simulink model "Hydrogen_platform"  (R2024b)
settings: Solver=VariableStepAuto  StartTime=0.0  StopTime=10.0  FixedStep=0.001  RelTol=1e-3
(part 1 of 2)
settings Model: Creator=Administrator  LastModifiedBy=wangx
settings OptimizationCC: DefaultParameterBehavior=Inlined  EnhancedBackFolding=on  PassReuseOutputArgsAs=Individual arguments  ZeroExternalMemoryAtStartup=off  ZeroInternalMemoryAtStartup=off  OptimizeBlockOrder=speed  DifferentSizesBufferReuse=on  OptimizationCustomize=off  EfficientTunableParamExpr=on
settings DebuggingCC: ParameterTunabilityLossMsg=error  ForceCombineOutputUpdateInSim=on
settings HardwareCC: TargetBitPerPointer=64  TargetBitPerSizeT=64  TargetBitPerPtrDiffT=64  TargetLongLongMode=on  TargetIntDivRoundTo=Zero  TargetEndianess=LittleEndian  TargetWordSize=64  TargetHWDeviceType=MATLAB Host  ProdEqTarget=off
settings ModelReferenceCC: EnableRefExpFcnMdlSchedulingChecks=on
settings SFSimCC: MATLABDynamicMemAlloc=off
settings RTWCC: Description=Embedded Coder  SystemTargetFile=ert.tlc  TemplateMakefile=ert_default_tmf  GPUComputeCapability=3.5
settings CodeAppCC: ForceParamTrailComments=on  IgnoreCustomStorageClasses=off  OperatorAnnotations=on  SimulinkDataObjDesc=on  SFDataObjDesc=on  InsertBlockDesc=on
settings ERTTargetCC: TargetLangStandard=C99 (ISO)  GenerateSampleERTMain=on  SupportContinuousTime=on  ERTCustomFileTemplate=example_file_process.tlc  DynamicArrayContainerType=coder::array

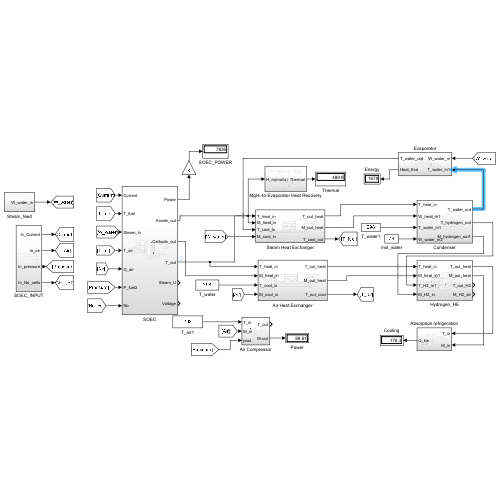
[thumbnail: Simulink's stored preview of the top-level diagram]
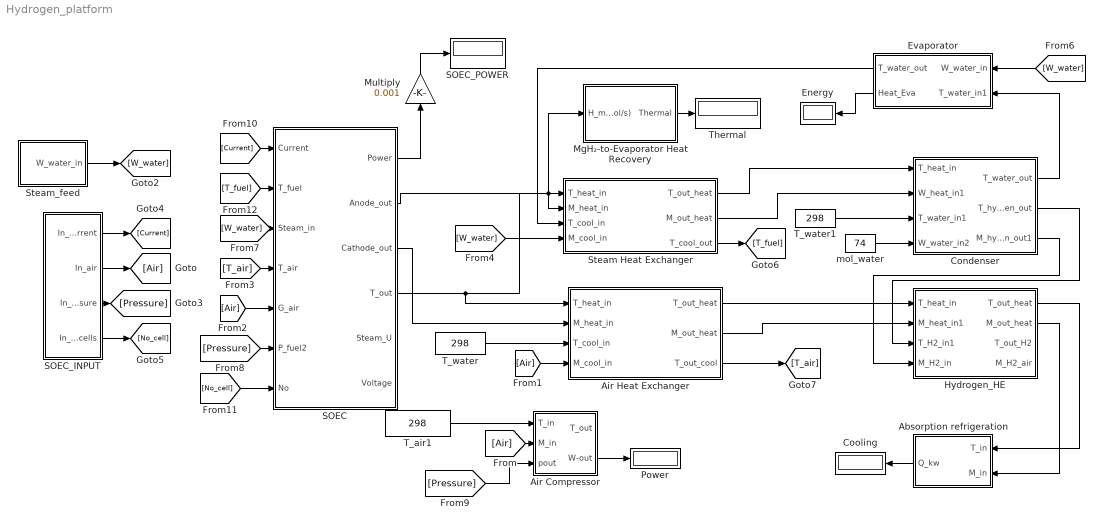
== system Hydrogen_platform ==
  Absorption refrigeration : Subsystem
  Air Compressor : Subsystem
  Air Heat Exchanger : Subsystem
  Condenser : Subsystem
  Cooling : Display
  Energy : Display
  Evaporator : Subsystem
  Hydrogen_HE : Subsystem
  MgH₂-to-Evaporator Heat Recovery : Subsystem
  Multiply : Gain  Gain=0.001
  Power : Display
  SOEC : Subsystem
  SOEC_INPUT : Subsystem
  SOEC_POWER : Display
  Steam Heat Exchanger : Subsystem
  Steam_feed : Subsystem
  T_air1 : Constant  Value=298
  T_water : Constant  Value=298
  T_water1 : Constant  Value=298
  Thermal : Display
  mol_water : Constant  Value=74
  wires:
  mol_water/1 -> Condenser/4(W_water_in2)
  SOEC/3(Cathode_out) -> Air Heat Exchanger/2(M_heat_in)
  T_air1/1 -> Air Compressor/1(T_in)
  SOEC/4(T_out) -> Steam Heat Exchanger/1(T_heat_in), Air Heat Exchanger/1(T_heat_in)
  Evaporator/1(T_water_out) -> Steam Heat Exchanger/3(T_cool_in)
  Condenser/1(T_water_out) -> Evaporator/2(T_water_in1)
  SOEC/2(Anode_out) -> MgH₂-to-Evaporator Heat Recovery/1(H_m(mol/s)), Steam Heat Exchanger/2(M_heat_in)
  [Air] -> Air Compressor/2(M_in)
  [Air] -> SOEC/5(G_air)
  SOEC_INPUT/2(In_air) -> [Air]
  [T_air] -> SOEC/4(T_air)
  [W_water] -> Steam Heat Exchanger/4(M_cool_in)
  Steam_feed/1(W_water_in) -> [W_water]
  [W_water] -> SOEC/3(Steam_in)
  SOEC_INPUT/3(In_pressure) -> [Pressure]
  [Pressure] -> SOEC/6(P_fuel2)
  [Pressure] -> Air Compressor/3(pout)
  SOEC_INPUT/1(In_Current) -> [Current]
  [Current] -> SOEC/1(Current)
  [No_cell] -> SOEC/7(No)
  SOEC_INPUT/4(In_No_cells) -> [No_cell]
  [T_fuel] -> SOEC/2(T_fuel)
  T_water1/1 -> Condenser/3(T_water_in1)
  Condenser/2(T_hydrogen_out) -> Hydrogen_HE/3(T_H2_in1)
  Condenser/3(M_hydrogen_out1) -> Hydrogen_HE/4(M_H2_in)
  Hydrogen_HE/1(T_out_heat) -> Absorption refrigeration/1(T_in)
  Hydrogen_HE/2(M_out_heat) -> Absorption refrigeration/2(M_in)
  Multiply/1 -> SOEC_POWER/1
  SOEC/1(Power) -> Multiply/1
  Evaporator/2(Heat_Eva) -> Energy/1
  Air Compressor/2(W-out) -> Power/1
  Steam Heat Exchanger/1(T_out_heat) -> Condenser/1(T_heat_in)
  Steam Heat Exchanger/2(M_out_heat) -> Condenser/2(W_heat_in1)
  Steam Heat Exchanger/3(T_cool_out) -> [T_fuel]
  [Air] -> Air Heat Exchanger/4(M_cool_in)
  T_water/1 -> Air Heat Exchanger/3(T_cool_in)
  Air Heat Exchanger/3(T_out_cool) -> [T_air]
  Air Heat Exchanger/1(T_out_heat) -> Hydrogen_HE/1(T_heat_in)
  Air Heat Exchanger/2(M_out_heat) -> Hydrogen_HE/2(M_heat_in1)
  [W_water] -> Evaporator/1(W_water_in)
  Absorption refrigeration/1(Q_kw) -> Cooling/1
  MgH₂-to-Evaporator Heat Recovery/1(Thermal) -> Thermal/1

== system Hydrogen_platform/Absorption refrigeration ==
  T_in : Inport
  M_in : Inport  Port=2
  Add : Sum  Inputs=-+
  Cop : Constant  Value=1.3
  Demux : Demux  Outputs=2
  Divide : Product  Inputs=**
  Energy : Product  Inputs=***
  Energy1 : Product  Inputs=***
  T_out : Constant  Value=273+120
  air_out1 : Subsystem
  air_out2 : Subsystem
  kW : Gain  Gain=0.001
  sum : Fcn  Expr=u(1)+u(2)
  Q_kw : Outport
  wires:
  M_in/1 -> sum/1, Demux/1
  Demux/1 -> air_out2/2(O2), air_out1/2(O2)
  Demux/2 -> air_out2/3(N2), air_out1/3(N2)
  T_in/1 -> Energy/2, air_out2/1(T_cool_out)
  air_out2/1(C_p) -> Energy/3
  Energy/1 -> Add/2
  sum/1 -> Energy1/2, Energy/1
  T_out/1 -> Energy1/1, air_out1/1(T_cool_out)
  air_out1/1(C_p) -> Energy1/3
  Energy1/1 -> Add/1
  Add/1 -> Divide/1
  Cop/1 -> Divide/2
  Divide/1 -> kW/1
  kW/1 -> Q_kw/1

== system Hydrogen_platform/Air Compressor ==
  T_in : Inport
  M_in : Inport  Port=2
  pout : Inport  Port=3
  Add : Sum  Inputs=+-
  Gain : Gain  Gain=1e-5
  Gain1 : Gain  Gain=0.21
  Gain2 : Gain  Gain=0.79
  Gain3 : Gain  Gain=0.001
  Mux : Mux  Inputs=2
  Product : Product
  Product1 : Product
  Product2 : Product
  T_jisuan : Fcn  Expr=u(1)*(1+(1/0.85)*(u(2)^0.285-1))
  air_out1 : Subsystem
  air_out3 : Subsystem
  T_out : Outport
  W-out : Outport  Port=2
  wires:
  T_jisuan/1 -> air_out1/1(T_cool_out), T_out/1, Product1/1
  Mux/1 -> T_jisuan/1
  T_in/1 -> air_out3/1(T_cool_out), Product/1, Mux/1
  pout/1 -> Gain/1
  Gain/1 -> Mux/2
  M_in/1 -> Product2/2, Gain2/1, Gain1/1
  Gain1/1 -> air_out1/2(O2), air_out3/2(O2)
  Gain2/1 -> air_out3/3(N2), air_out1/3(N2)
  air_out3/1(C_p) -> Product/2
  air_out1/1(C_p) -> Product1/2
  Product1/1 -> Add/1
  Product/1 -> Add/2
  Product2/1 -> Gain3/1
  Add/1 -> Product2/1
  Gain3/1 -> W-out/1

== system Hydrogen_platform/Air Heat Exchanger ==
  T_heat_in : Inport
  M_heat_in : Inport  Port=2
  T_cool_in : Inport  Port=3
  M_cool_in : Inport  Port=4
  First_Air_HE : Subsystem
  Second_Air_HE : Subsystem
  T_out_heat : Outport
  M_out_heat : Outport  Port=2
  T_out_cool : Outport  Port=3
  wires:
  First_Air_HE/1(T_out_heat) -> Second_Air_HE/1(T_heat_in)
  First_Air_HE/2(M_out_heat) -> Second_Air_HE/2(M_heat_in1)
  Second_Air_HE/3(T_out_cool) -> First_Air_HE/3(T_cool_in1)
  Second_Air_HE/4(M_out_cool) -> First_Air_HE/4(M_cool_in)
  M_cool_in/1 -> Second_Air_HE/4(M_cool_in)
  First_Air_HE/3(T_out_cool) -> T_out_cool/1
  T_cool_in/1 -> Second_Air_HE/3(T_cool_in1)
  T_heat_in/1 -> First_Air_HE/1(T_heat_in)
  M_heat_in/1 -> First_Air_HE/2(M_heat_in1)
  Second_Air_HE/1(T_out_heat) -> T_out_heat/1
  Second_Air_HE/2(M_out_heat) -> M_out_heat/1

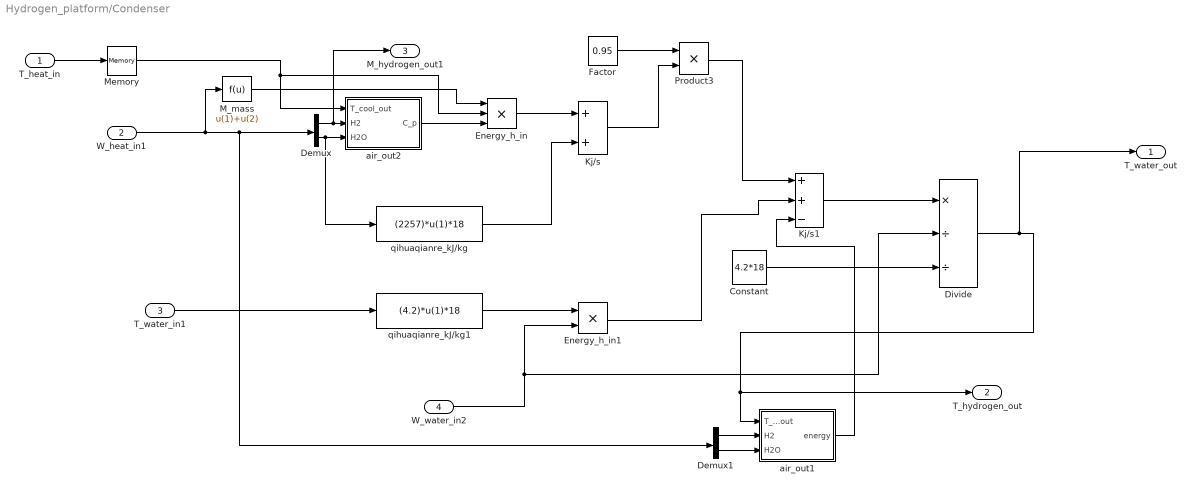
== system Hydrogen_platform/Condenser ==
  T_heat_in : Inport
  W_heat_in1 : Inport  Port=2
  T_water_in1 : Inport  Port=3
  W_water_in2 : Inport  Port=4
  Constant : Constant  Value=4.2*18
  Demux : Demux  Outputs=2
  Demux1 : Demux  Outputs=2
  Divide : Product  Inputs=*//
  Energy_h_in : Product  Inputs=3
  Energy_h_in1 : Product
  Factor : Constant  Value=0.95
  Kj/s : Sum
  Kj/s1 : Sum  Inputs=++-
  M_mass : Fcn  Expr=u(1)+u(2)
  Memory : Memory  InitialCondition=500
  Product3 : Product
  air_out1 : Subsystem
  air_out2 : Subsystem
  qihuaqianre_kJ/kg : Fcn  Expr=(2257)*u(1)*18
  qihuaqianre_kJ/kg1 : Fcn  Expr=(4.2)*u(1)*18
  T_water_out : Outport
  T_hydrogen_out : Outport  Port=2
  M_hydrogen_out1 : Outport  Port=3
  wires:
  Demux/1 -> M_hydrogen_out1/1, air_out2/2(H2)
  Demux/2 -> qihuaqianre_kJ/kg/1, air_out2/3(H2O)
  W_heat_in1/1 -> M_mass/1, Demux/1, Demux1/1
  T_heat_in/1 -> Memory/1
  air_out2/1(C_p) -> Energy_h_in/3
  M_mass/1 -> Energy_h_in/1
  Energy_h_in/1 -> Kj/s/1
  Factor/1 -> Product3/1
  Kj/s/1 -> Product3/2
  qihuaqianre_kJ/kg/1 -> Kj/s/2
  T_water_in1/1 -> qihuaqianre_kJ/kg1/1
  qihuaqianre_kJ/kg1/1 -> Energy_h_in1/1
  W_water_in2/1 -> Divide/2, Energy_h_in1/2
  Product3/1 -> Kj/s1/1
  Energy_h_in1/1 -> Kj/s1/2
  Constant/1 -> Divide/3
  Divide/1 -> T_water_out/1, air_out1/1(T_cool_out), T_hydrogen_out/1
  Demux1/1 -> air_out1/2(H2)
  Demux1/2 -> air_out1/3(H2O)
  air_out1/1(energy) -> Kj/s1/3
  Kj/s1/1 -> Divide/1
  Memory/1 -> air_out2/1(T_cool_out), Energy_h_in/2

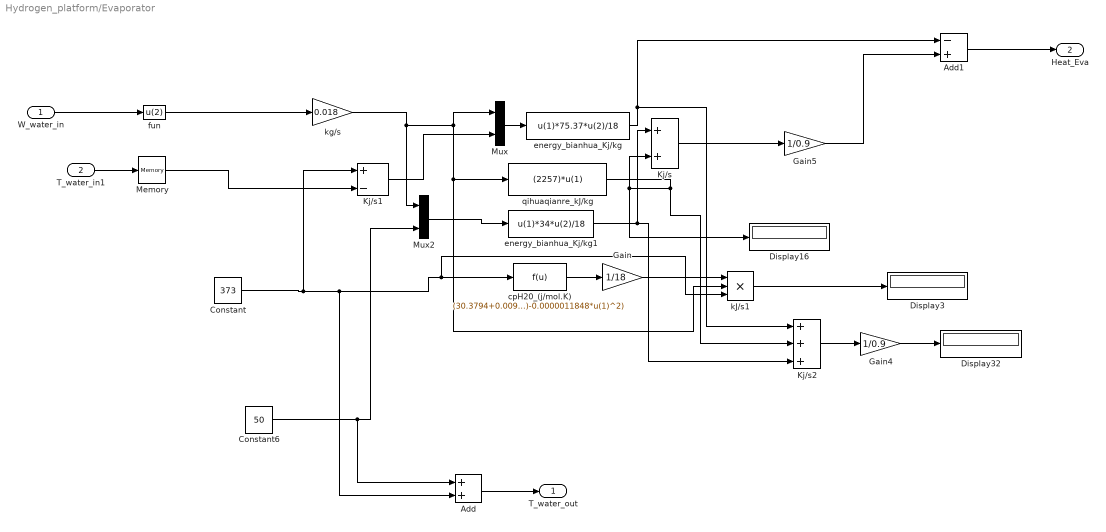
== system Hydrogen_platform/Evaporator ==
  W_water_in : Inport
  T_water_in1 : Inport  Port=2
  Add : Sum
  Add1 : Sum  Inputs=-+
  Constant : Constant  Value=373
  Constant6 : Constant  Value=50
  Display16 : Display
  Display3 : Display
  Display32 : Display
  Gain : Gain  Gain=1/18
  Gain4 : Gain  Gain=1/0.9
  Gain5 : Gain  Gain=1/0.9
  Kj/s : Sum
  Kj/s1 : Sum  Inputs=+-
  Kj/s2 : Sum  Inputs=+++
  Memory : Memory  InitialCondition=300
  Mux : Mux  Inputs=2
  Mux2 : Mux  Inputs=2
  cpH20_(j/mol.K) : Fcn  Expr=(30.3794+0.0096212*u(1)-0.0000011848*u(1)^2)
  energy_bianhua_Kj/kg : Fcn  Expr=u(1)*75.37*u(2)/18
  energy_bianhua_Kj/kg1 : Fcn  Expr=u(1)*34*u(2)/18
  fun : Fcn  Expr=u(2)
  kJ/s1 : Product  Inputs=3
  kg/s : Gain  Gain=0.018
  qihuaqianre_kJ/kg : Fcn  Expr=(2257)*u(1)
  T_water_out : Outport
  Heat_Eva : Outport  Port=2
  wires:
  W_water_in/1 -> fun/1
  energy_bianhua_Kj/kg/1 -> Kj/s2/1, Add1/1
  qihuaqianre_kJ/kg/1 -> Kj/s2/2, Kj/s/2, Display16/1
  Constant/1 -> kJ/s1/3, cpH20_(j/mol.K)/1, Add/2, Kj/s1/1
  cpH20_(j/mol.K)/1 -> Gain/1
  Gain/1 -> kJ/s1/1
  kJ/s1/1 -> Display3/1
  T_water_in1/1 -> Memory/1
  Mux/1 -> energy_bianhua_Kj/kg/1
  Kj/s1/1 -> Mux/2
  Memory/1 -> Kj/s1/2
  energy_bianhua_Kj/kg1/1 -> Kj/s2/3, Kj/s/1
  kg/s/1 -> Mux2/1, Mux/1, kJ/s1/2, qihuaqianre_kJ/kg/1
  Mux2/1 -> energy_bianhua_Kj/kg1/1
  Constant6/1 -> Add/1, Mux2/2
  Add/1 -> T_water_out/1
  Kj/s/1 -> Gain5/1
  Kj/s2/1 -> Gain4/1
  Gain4/1 -> Display32/1
  Gain5/1 -> Add1/2
  fun/1 -> kg/s/1
  Add1/1 -> Heat_Eva/1

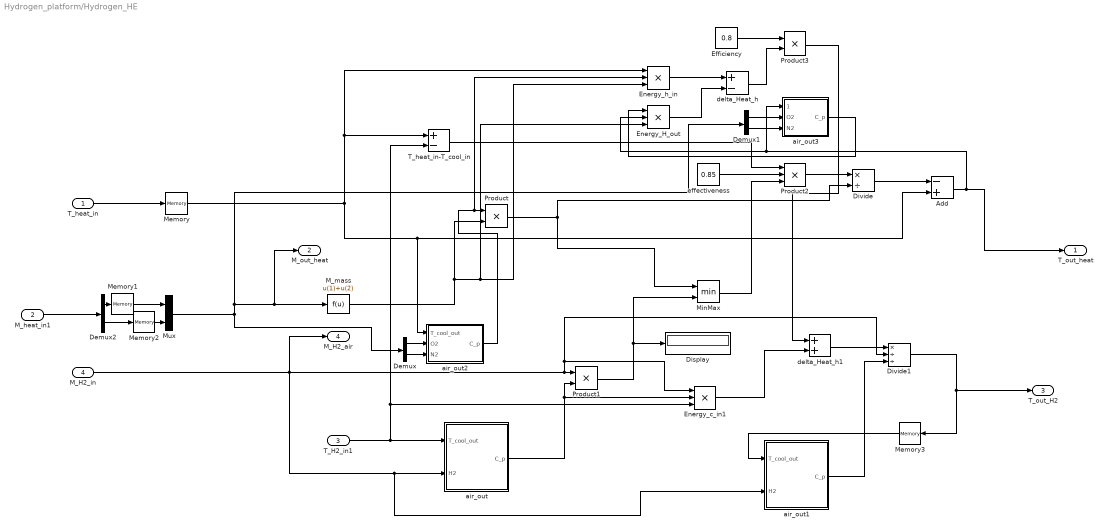
== system Hydrogen_platform/Hydrogen_HE ==
  T_heat_in : Inport
  M_heat_in1 : Inport  Port=2
  T_H2_in1 : Inport  Port=3
  M_H2_in : Inport  Port=4
  Add : Sum  Inputs=-+
  Demux : Demux  Outputs=2
  Demux1 : Demux  Outputs=2
  Demux2 : Demux  Outputs=2
  Display : Display
  Divide : Product  Inputs=*/
  Divide1 : Product  Inputs=*//
  Efficiency : Constant  Value=0.8
  Energy_H_out : Product  Inputs=3
  Energy_c_in1 : Product  Inputs=3
  Energy_h_in : Product  Inputs=3
  M_mass : Fcn  Expr=u(1)+u(2)
  Memory : Memory  InitialCondition=800
  Memory1 : Memory  InitialCondition=3
  Memory2 : Memory  InitialCondition=3
  Memory3 : Memory  InitialCondition=400
  MinMax : MinMax  Inputs=2
  Mux : Mux  Inputs=2
  Product : Product
  Product1 : Product
  Product2 : Product  Inputs=3
  Product3 : Product
  T_heat_in-T_cool_in : Sum  Inputs=+-
  air_out : Subsystem
  air_out1 : Subsystem
  air_out2 : Subsystem
  air_out3 : Subsystem
  delta_Heat_h : Sum  Inputs=+-
  delta_Heat_h1 : Sum
  effectiveness : Constant  Value=0.85
  T_out_heat : Outport
  M_out_heat : Outport  Port=2
  T_out_H2 : Outport  Port=3
  M_H2_air : Outport  Port=4
  wires:
  Mux/1 -> M_out_heat/1, M_mass/1, Demux1/1, Demux/1
  Product2/1 -> Divide/1
  T_heat_in/1 -> Memory/1
  MinMax/1 -> Product2/3
  M_H2_in/1 -> M_H2_air/1, Energy_c_in1/1, Divide1/2, Product1/1, air_out1/2(H2), air_out/2(H2)
  air_out/1(C_p) -> Product1/2, Energy_c_in1/2
  T_H2_in1/1 -> Energy_c_in1/3, T_heat_in-T_cool_in/2, air_out/1(T_cool_out)
  T_heat_in-T_cool_in/1 -> Product2/1
  air_out2/1(C_p) -> Product/1, Energy_h_in/2
  effectiveness/1 -> Product2/2
  Energy_H_out/1 -> delta_Heat_h/2
  Product1/1 -> MinMax/2, Display/1
  Product/1 -> MinMax/1, Divide/2
  Add/1 -> air_out3/1(T_cool_out), Energy_H_out/2, T_out_heat/1
  Divide/1 -> Add/1
  Energy_h_in/1 -> delta_Heat_h/1
  Energy_c_in1/1 -> delta_Heat_h1/2
  delta_Heat_h1/1 -> Divide1/1
  air_out1/1(C_p) -> Divide1/3
  Divide1/1 -> Memory3/1, T_out_H2/1
  delta_Heat_h/1 -> Product3/2
  Product3/1 -> delta_Heat_h1/1
  Efficiency/1 -> Product3/1
  M_mass/1 -> Energy_h_in/3, Energy_H_out/3, Product/2
  Demux/1 -> air_out2/2(O2)
  Demux/2 -> air_out2/3(N2)
  Demux1/1 -> air_out3/2(O2)
  Demux1/2 -> air_out3/3(N2)
  air_out3/1(C_p) -> Energy_H_out/1
  Memory/1 -> Energy_h_in/1, T_heat_in-T_cool_in/1, air_out2/1(T_cool_out), Add/2
  Demux2/2 -> Memory2/1
  Memory2/1 -> Mux/2
  Memory1/1 -> Mux/1
  Demux2/1 -> Memory1/1
  M_heat_in1/1 -> Demux2/1
  Memory3/1 -> air_out1/1(T_cool_out)

== system Hydrogen_platform/MgH₂-to-Evaporator Heat Recovery ==
  H_m(mol/s) : Inport
  Divide : Product  Inputs=*/*
  H2_kg : Fcn  Expr=u(1)*2*3600/1000
  KgH2/Tank : Constant  Value=25
  kWh/tank : Constant  Value=61.18
  kg/hour : Display
  Thermal : Outport
  wires:
  H_m(mol/s)/1 -> H2_kg/1
  H2_kg/1 -> Divide/1, kg/hour/1
  KgH2/Tank/1 -> Divide/2
  kWh/tank/1 -> Divide/3
  Divide/1 -> Thermal/1

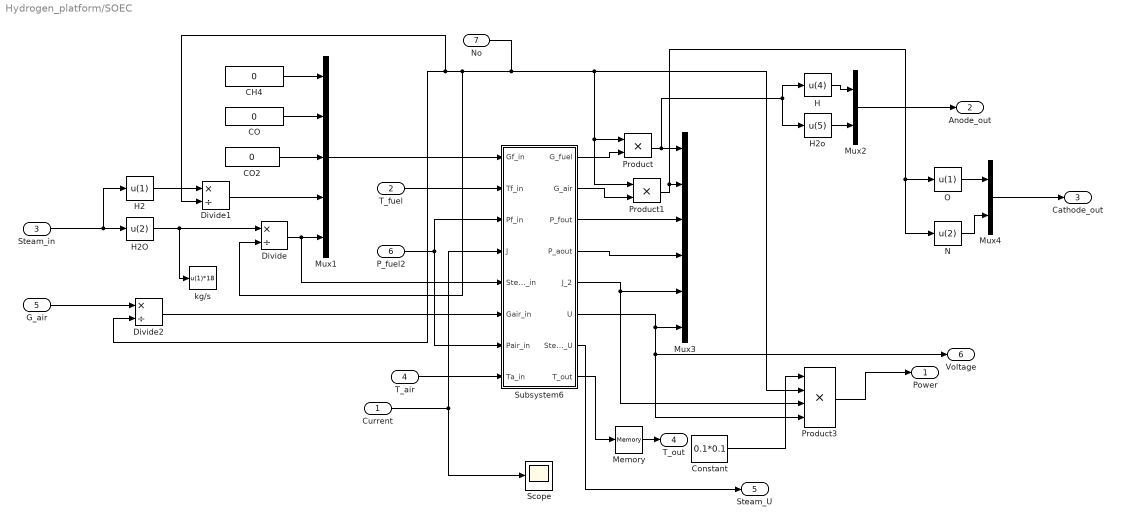
== system Hydrogen_platform/SOEC ==
  Current : Inport
  T_fuel : Inport  Port=2
  Steam_in : Inport  Port=3
  T_air : Inport  Port=4
  G_air : Inport  Port=5
  P_fuel2 : Inport  Port=6
  No : Inport  Port=7
  CH4 : Constant  Value=0
  CO : Constant  Value=0
  CO2 : Constant  Value=0
  Constant : Constant  Value=0.1*0.1
  Divide : Product  Inputs=*/
  Divide1 : Product  Inputs=*/
  Divide2 : Product  Inputs=*/
  H : Fcn  Expr=u(4)
  H2 : Fcn  Expr=u(1)
  H2O : Fcn  Expr=u(2)
  H2o : Fcn  Expr=u(5)
  Memory : Memory  InitialCondition=800
  Mux1 : Mux  Inputs=5
  Mux2 : Mux  Inputs=2
  Mux3 : Mux  Inputs=6
  Mux4 : Mux  Inputs=2
  N : Fcn  Expr=u(2)
  O : Fcn  Expr=u(1)
  Product : Product
  Product1 : Product
  Product3 : Product  Inputs=4
  Scope : Scope
  Subsystem6 : Subsystem
  kg/s : Fcn  Expr=u(1)*18
  Power : Outport
  Anode_out : Outport  Port=2
  Cathode_out : Outport  Port=3
  T_out : Outport  Port=4
  Steam_U : Outport  Port=5
  Voltage : Outport  Port=6
  wires:
  Subsystem6/8(T_out) -> Memory/1
  T_fuel/1 -> Subsystem6/2(Tf_in)
  Current/1 -> Subsystem6/4(J), Scope/1
  Product/1 -> H/1, H2o/1, Mux3/1
  Mux2/1 -> Anode_out/1
  H/1 -> Mux2/1
  Subsystem6/2("\tG_air") -> Product1/2
  No/1 -> Divide2/2, Divide1/2, Divide/2, Product3/2, Product/1, Product1/1
  Subsystem6/5(J_2) -> Mux3/5, Product3/3
  P_fuel2/1 -> Subsystem6/3(Pf_in), Subsystem6/7(Pair_in)
  CO2/1 -> Mux1/3
  Subsystem6/6(U) -> Product3/4, Voltage/1, Mux3/6
  Mux1/1 -> Subsystem6/1(Gf_in)
  Subsystem6/4("\tP_aout") -> Mux3/4
  Product1/1 -> N/1, O/1, Mux3/2
  CH4/1 -> Mux1/1
  CO/1 -> Mux1/2
  H2o/1 -> Mux2/2
  Product3/1 -> Power/1
  Subsystem6/3("\tP_fout") -> Mux3/3
  Constant/1 -> Product3/1
  Subsystem6/1("\tG_fuel") -> Product/2
  Divide/1 -> Mux1/5, Subsystem6/5(Steam_in)
  Subsystem6/7(Steam_U) -> Steam_U/1
  Divide1/1 -> Mux1/4
  Steam_in/1 -> H2O/1, H2/1
  T_air/1 -> Subsystem6/8(Ta_in)
  Divide2/1 -> Subsystem6/6(Gair_in)
  G_air/1 -> Divide2/1
  O/1 -> Mux4/1
  N/1 -> Mux4/2
  Mux4/1 -> Cathode_out/1
  H2/1 -> Divide1/1
  H2O/1 -> kg/s/1, Divide/1
  Memory/1 -> T_out/1

== system Hydrogen_platform/SOEC_INPUT ==
  Air_in : Constant  Value=37
  Current : Constant  Value=5000
  No_fc : Constant  Value=107300
  P_f : Constant  Value=2e5
  In_Current : Outport
  In_air : Outport  Port=2
  In_pressure : Outport  Port=3
  In_No_cells : Outport  Port=4
  wires:
  Current/1 -> In_Current/1
  Air_in/1 -> In_air/1
  P_f/1 -> In_pressure/1
  No_fc/1 -> In_No_cells/1

== system Hydrogen_platform/Steam Heat Exchanger ==
  T_heat_in : Inport
  M_heat_in : Inport  Port=2
  T_cool_in : Inport  Port=3
  M_cool_in : Inport  Port=4
  First_steam_HE : Subsystem
  Second_steam_HE : Subsystem
  T_out_heat : Outport
  M_out_heat : Outport  Port=2
  T_cool_out : Outport  Port=3
  wires:
  T_heat_in/1 -> First_steam_HE/1(T_heat_in)
  M_heat_in/1 -> First_steam_HE/2(M_heat_in1)
  M_cool_in/1 -> Second_steam_HE/4(M_cool_in), First_steam_HE/4(M_cool_in)
  Second_steam_HE/1(T_out_heat) -> T_out_heat/1
  Second_steam_HE/2(M_out_heat) -> M_out_heat/1
  T_cool_in/1 -> Second_steam_HE/3(T_cool_in1)
  First_steam_HE/1(T_out_heat) -> Second_steam_HE/1(T_heat_in)
  First_steam_HE/2(M_out_heat) -> Second_steam_HE/2(M_heat_in1)
  First_steam_HE/3(T_out_cool) -> T_cool_out/1
  Second_steam_HE/3(T_out_cool) -> First_steam_HE/3(T_cool_in1)

== system Hydrogen_platform/Steam_feed ==
  Display : Display
  Gain2 : Gain
  H2 : Constant  Value=0
  H2O : Constant
  Mux : Mux  Inputs=2
  Product : Product
  Product1 : Product
  Steam_in : Constant  Value=37
  xxx : Gain
  W_water_in : Outport
  wires:
  H2/1 -> Product/1
  H2O/1 -> Product1/2
  Gain2/1 -> xxx/1
  Steam_in/1 -> Gain2/1
  xxx/1 -> Product1/1, Product/2
  Product1/1 -> Mux/2
  Product/1 -> Mux/1
  Mux/1 -> Display/1, W_water_in/1

== system Hydrogen_platform/Absorption refrigeration/air_out1 ==
  T_cool_out : Inport
  O2 : Inport  Port=2
  N2 : Inport  Port=3
  Add : Sum
  Add1 : Sum
  Divide : Product  Inputs=*/
  Product4 : Product
  Product5 : Product
  cpN2_T : Fcn  Expr=(27.32+(6.226*10^(-3))*u(1)-(9.502*10^(-7))*u(1)^2)
  cpO2_T : Fcn  Expr=(25.8911+0.01299*u(1)-0.0000038644*u(1)^2)
  C_p : Outport  VectorParamsAs1DForOutWhenUnconnected=off
  wires:
  T_cool_out/1 -> cpO2_T/1, cpN2_T/1
  cpN2_T/1 -> Product4/1
  N2/1 -> Add1/1, Product4/2
  cpO2_T/1 -> Product5/1
  O2/1 -> Add1/2, Product5/2
  Product4/1 -> Add/1
  Product5/1 -> Add/2
  Add/1 -> Divide/1
  Add1/1 -> Divide/2
  Divide/1 -> C_p/1

== system Hydrogen_platform/Absorption refrigeration/air_out2 ==
  T_cool_out : Inport
  O2 : Inport  Port=2
  N2 : Inport  Port=3
  Add : Sum
  Add1 : Sum
  Divide : Product  Inputs=*/
  Product4 : Product
  Product5 : Product
  cpN2_T : Fcn  Expr=(27.32+(6.226*10^(-3))*u(1)-(9.502*10^(-7))*u(1)^2)
  cpO2_T : Fcn  Expr=(25.8911+0.01299*u(1)-0.0000038644*u(1)^2)
  C_p : Outport  VectorParamsAs1DForOutWhenUnconnected=off
  wires:
  T_cool_out/1 -> cpO2_T/1, cpN2_T/1
  cpN2_T/1 -> Product4/1
  N2/1 -> Add1/1, Product4/2
  cpO2_T/1 -> Product5/1
  O2/1 -> Add1/2, Product5/2
  Product4/1 -> Add/1
  Product5/1 -> Add/2
  Add/1 -> Divide/1
  Add1/1 -> Divide/2
  Divide/1 -> C_p/1

== system Hydrogen_platform/Air Compressor/air_out1 ==
  T_cool_out : Inport
  O2 : Inport  Port=2
  N2 : Inport  Port=3
  Add : Sum
  Add1 : Sum
  Divide : Product  Inputs=*/
  Product4 : Product
  Product5 : Product
  cpN2_T : Fcn  Expr=(27.32+(6.226*10^(-3))*u(1)-(9.502*10^(-7))*u(1)^2)
  cpO2_T : Fcn  Expr=(25.8911+0.01299*u(1)-0.0000038644*u(1)^2)
  C_p : Outport  VectorParamsAs1DForOutWhenUnconnected=off
  wires:
  T_cool_out/1 -> cpO2_T/1, cpN2_T/1
  cpN2_T/1 -> Product4/1
  N2/1 -> Add1/1, Product4/2
  cpO2_T/1 -> Product5/1
  O2/1 -> Add1/2, Product5/2
  Product4/1 -> Add/1
  Product5/1 -> Add/2
  Add/1 -> Divide/1
  Add1/1 -> Divide/2
  Divide/1 -> C_p/1

== system Hydrogen_platform/Air Compressor/air_out3 ==
  T_cool_out : Inport
  O2 : Inport  Port=2
  N2 : Inport  Port=3
  Add : Sum
  Add1 : Sum
  Divide : Product  Inputs=*/
  Product4 : Product
  Product5 : Product
  cpN2_T : Fcn  Expr=(27.32+(6.226*10^(-3))*u(1)-(9.502*10^(-7))*u(1)^2)
  cpO2_T : Fcn  Expr=(25.8911+0.01299*u(1)-0.0000038644*u(1)^2)
  C_p : Outport  VectorParamsAs1DForOutWhenUnconnected=off
  wires:
  T_cool_out/1 -> cpO2_T/1, cpN2_T/1
  cpN2_T/1 -> Product4/1
  N2/1 -> Add1/1, Product4/2
  cpO2_T/1 -> Product5/1
  O2/1 -> Add1/2, Product5/2
  Product4/1 -> Add/1
  Product5/1 -> Add/2
  Add/1 -> Divide/1
  Add1/1 -> Divide/2
  Divide/1 -> C_p/1

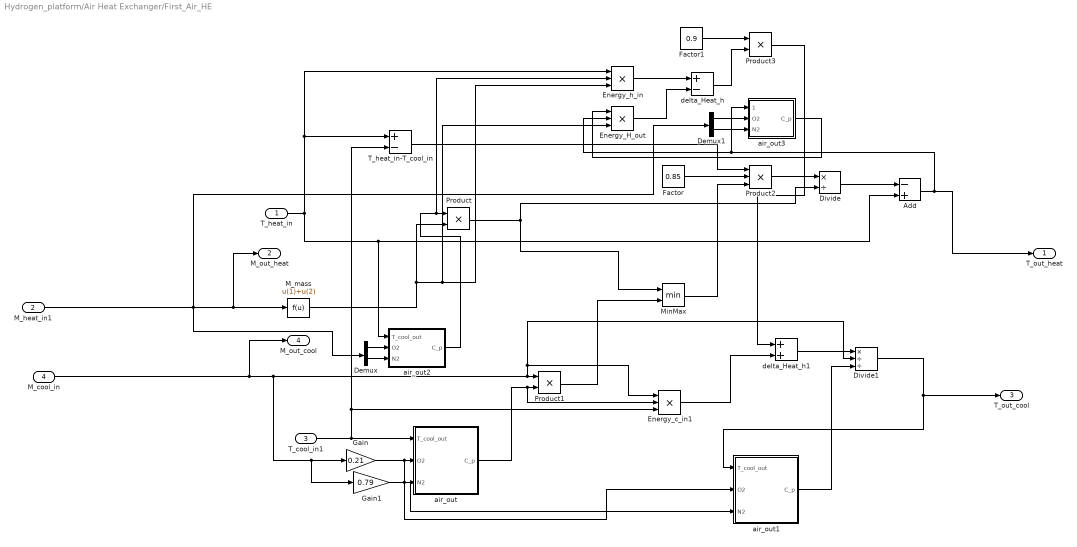
== system Hydrogen_platform/Air Heat Exchanger/First_Air_HE ==
  T_heat_in : Inport
  M_heat_in1 : Inport  Port=2
  T_cool_in1 : Inport  Port=3
  M_cool_in : Inport  Port=4
  Add : Sum  Inputs=-+
  Demux : Demux  Outputs=2
  Demux1 : Demux  Outputs=2
  Divide : Product  Inputs=*/
  Divide1 : Product  Inputs=*//
  Energy_H_out : Product  Inputs=3
  Energy_c_in1 : Product  Inputs=3
  Energy_h_in : Product  Inputs=3
  Factor : Constant  Value=0.85
  Factor1 : Constant  Value=0.9
  Gain : Gain  Gain=0.21
  Gain1 : Gain  Gain=0.79
  M_mass : Fcn  Expr=u(1)+u(2)
  MinMax : MinMax  Inputs=2
  Product : Product
  Product1 : Product
  Product2 : Product  Inputs=3
  Product3 : Product
  T_heat_in-T_cool_in : Sum  Inputs=+-
  air_out : Subsystem
  air_out1 : Subsystem
  air_out2 : Subsystem
  air_out3 : Subsystem
  delta_Heat_h : Sum  Inputs=+-
  delta_Heat_h1 : Sum
  T_out_heat : Outport
  M_out_heat : Outport  Port=2
  T_out_cool : Outport  Port=3
  M_out_cool : Outport  Port=4
  wires:
  M_heat_in1/1 -> Demux1/1, Demux/1, M_out_heat/1, M_mass/1
  Product2/1 -> Divide/1
  T_heat_in/1 -> air_out2/1(T_cool_out), Add/2, Energy_h_in/1, T_heat_in-T_cool_in/1
  MinMax/1 -> Product2/3
  M_cool_in/1 -> M_out_cool/1, Energy_c_in1/1, Divide1/2, Product1/1, Gain1/1, Gain/1
  air_out/1(C_p) -> Energy_c_in1/2, Product1/2
  T_cool_in1/1 -> Energy_c_in1/3, T_heat_in-T_cool_in/2, air_out/1(T_cool_out)
  Gain/1 -> air_out1/2(O2), air_out/2(O2)
  T_heat_in-T_cool_in/1 -> Product2/1
  air_out2/1(C_p) -> Product/1, Energy_h_in/2
  Factor/1 -> Product2/2
  Energy_H_out/1 -> delta_Heat_h/2
  Product1/1 -> MinMax/2
  Product/1 -> MinMax/1, Divide/2
  Add/1 -> air_out3/1(T_cool_out), Energy_H_out/2, T_out_heat/1
  Gain1/1 -> air_out1/3(N2), air_out/3(N2)
  Divide/1 -> Add/1
  Energy_h_in/1 -> delta_Heat_h/1
  Energy_c_in1/1 -> delta_Heat_h1/2
  delta_Heat_h1/1 -> Divide1/1
  air_out1/1(C_p) -> Divide1/3
  Divide1/1 -> T_out_cool/1, air_out1/1(T_cool_out)
  delta_Heat_h/1 -> Product3/2
  Product3/1 -> delta_Heat_h1/1
  Factor1/1 -> Product3/1
  M_mass/1 -> Energy_h_in/3, Energy_H_out/3, Product/2
  Demux/1 -> air_out2/2(O2)
  Demux/2 -> air_out2/3(N2)
  Demux1/1 -> air_out3/2(O2)
  Demux1/2 -> air_out3/3(N2)
  air_out3/1(C_p) -> Energy_H_out/1

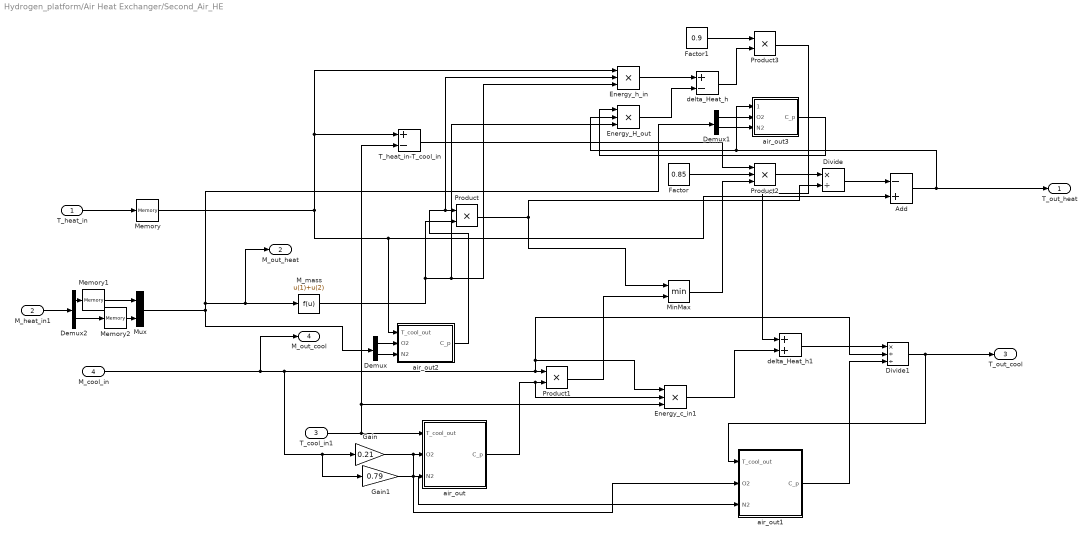
== system Hydrogen_platform/Air Heat Exchanger/Second_Air_HE ==
  T_heat_in : Inport
  M_heat_in1 : Inport  Port=2
  T_cool_in1 : Inport  Port=3
  M_cool_in : Inport  Port=4
  Add : Sum  Inputs=-+
  Demux : Demux  Outputs=2
  Demux1 : Demux  Outputs=2
  Demux2 : Demux  Outputs=2
  Divide : Product  Inputs=*/
  Divide1 : Product  Inputs=*//
  Energy_H_out : Product  Inputs=3
  Energy_c_in1 : Product  Inputs=3
  Energy_h_in : Product  Inputs=3
  Factor : Constant  Value=0.85
  Factor1 : Constant  Value=0.9
  Gain : Gain  Gain=0.21
  Gain1 : Gain  Gain=0.79
  M_mass : Fcn  Expr=u(1)+u(2)
  Memory : Memory  InitialCondition=800
  Memory1 : Memory  InitialCondition=3
  Memory2 : Memory  InitialCondition=3
  MinMax : MinMax  Inputs=2
  Mux : Mux  Inputs=2
  Product : Product
  Product1 : Product
  Product2 : Product  Inputs=3
  Product3 : Product
  T_heat_in-T_cool_in : Sum  Inputs=+-
  air_out : Subsystem
  air_out1 : Subsystem
  air_out2 : Subsystem
  air_out3 : Subsystem
  delta_Heat_h : Sum  Inputs=+-
  delta_Heat_h1 : Sum
  T_out_heat : Outport
  M_out_heat : Outport  Port=2
  T_out_cool : Outport  Port=3
  M_out_cool : Outport  Port=4
  wires:
  Mux/1 -> M_out_heat/1, M_mass/1, Demux1/1, Demux/1
  Product2/1 -> Divide/1
  MinMax/1 -> Product2/3
  M_cool_in/1 -> M_out_cool/1, Energy_c_in1/1, Divide1/2, Product1/1, Gain1/1, Gain/1
  air_out/1(C_p) -> Energy_c_in1/2, Product1/2
  T_cool_in1/1 -> T_heat_in-T_cool_in/2, Energy_c_in1/3, air_out/1(T_cool_out)
  Gain/1 -> air_out1/2(O2), air_out/2(O2)
  T_heat_in-T_cool_in/1 -> Product2/1
  air_out2/1(C_p) -> Product/1, Energy_h_in/2
  Factor/1 -> Product2/2
  Energy_H_out/1 -> delta_Heat_h/2
  Product1/1 -> MinMax/2
  Product/1 -> MinMax/1, Divide/2
  Add/1 -> air_out3/1(T_cool_out), Energy_H_out/2, T_out_heat/1
  Gain1/1 -> air_out1/3(N2), air_out/3(N2)
  Divide/1 -> Add/1
  Energy_h_in/1 -> delta_Heat_h/1
  Energy_c_in1/1 -> delta_Heat_h1/2
  delta_Heat_h1/1 -> Divide1/1
  air_out1/1(C_p) -> Divide1/3
  Divide1/1 -> air_out1/1(T_cool_out), T_out_cool/1
  delta_Heat_h/1 -> Product3/2
  Product3/1 -> delta_Heat_h1/1
  Factor1/1 -> Product3/1
  M_mass/1 -> Energy_h_in/3, Energy_H_out/3, Product/2
  Demux/1 -> air_out2/2(O2)
  Demux/2 -> air_out2/3(N2)
  Demux1/1 -> air_out3/2(O2)
  Demux1/2 -> air_out3/3(N2)
  air_out3/1(C_p) -> Energy_H_out/1
  Memory/1 -> Energy_h_in/1, T_heat_in-T_cool_in/1, air_out2/1(T_cool_out), Add/2
  M_heat_in1/1 -> Demux2/1
  Demux2/1 -> Memory1/1
  Demux2/2 -> Memory2/1
  Memory1/1 -> Mux/1
  Memory2/1 -> Mux/2
  T_heat_in/1 -> Memory/1

== system Hydrogen_platform/Condenser/air_out1 ==
  T_cool_out : Inport
  H2 : Inport  Port=2
  H2O : Inport  Port=3
  Add : Sum
  Constant : Constant  Value=4.2*18
  Memory : Memory  InitialCondition=500
  Product1 : Product
  Product4 : Product
  Product5 : Product
  cpH2_T : Fcn  Expr=(29.08-0.00084*u(1)+0.000002*u(1)^2)
  energy : Outport  VectorParamsAs1DForOutWhenUnconnected=off
  wires:
  T_cool_out/1 -> Memory/1
  Constant/1 -> Product4/1
  H2O/1 -> Product4/2
  cpH2_T/1 -> Product5/1
  H2/1 -> Product5/2
  Product4/1 -> Add/1
  Product5/1 -> Add/2
  Add/1 -> Product1/1
  Product1/1 -> energy/1
  Memory/1 -> Product1/2, cpH2_T/1

== system Hydrogen_platform/Condenser/air_out2 ==
  T_cool_out : Inport
  H2 : Inport  Port=2
  H2O : Inport  Port=3
  Add : Sum
  Add1 : Sum
  Divide : Product  Inputs=*/
  Product4 : Product
  Product5 : Product
  cpH20_T : Fcn  Expr=(30.3794+0.0096212*u(1)-0.0000011848*u(1)^2)
  cpH2_T : Fcn  Expr=(29.08-0.00084*u(1)+0.000002*u(1)^2)
  C_p : Outport  VectorParamsAs1DForOutWhenUnconnected=off
  wires:
  T_cool_out/1 -> cpH20_T/1, cpH2_T/1
  cpH20_T/1 -> Product4/1
  H2O/1 -> Add1/1, Product4/2
  cpH2_T/1 -> Product5/1
  H2/1 -> Add1/2, Product5/2
  Product4/1 -> Add/1
  Product5/1 -> Add/2
  Add/1 -> Divide/1
  Add1/1 -> Divide/2
  Divide/1 -> C_p/1

== system Hydrogen_platform/Hydrogen_HE/air_out ==
  T_cool_out : Inport
  H2 : Inport  Port=2
  Divide : Product  Inputs=*/
  Product4 : Product
  cpH2_T : Fcn  Expr=(29.08-0.00084*u(1)+0.000002*u(1)^2)
  C_p : Outport  VectorParamsAs1DForOutWhenUnconnected=off
  wires:
  T_cool_out/1 -> cpH2_T/1
  cpH2_T/1 -> Product4/1
  Product4/1 -> Divide/1
  Divide/1 -> C_p/1
  H2/1 -> Divide/2, Product4/2

== system Hydrogen_platform/Hydrogen_HE/air_out1 ==
  T_cool_out : Inport
  H2 : Inport  Port=2
  Divide : Product  Inputs=*/
  Product4 : Product
  cpH2_T : Fcn  Expr=(29.08-0.00084*u(1)+0.000002*u(1)^2)
  C_p : Outport  VectorParamsAs1DForOutWhenUnconnected=off
  wires:
  T_cool_out/1 -> cpH2_T/1
  cpH2_T/1 -> Product4/1
  Product4/1 -> Divide/1
  Divide/1 -> C_p/1
  H2/1 -> Divide/2, Product4/2

== system Hydrogen_platform/Hydrogen_HE/air_out2 ==
  T_cool_out : Inport
  O2 : Inport  Port=2
  N2 : Inport  Port=3
  Add : Sum
  Add1 : Sum
  Divide : Product  Inputs=*/
  Product4 : Product
  Product5 : Product
  cpN2_T : Fcn  Expr=(27.32+(6.226*10^(-3))*u(1)-(9.502*10^(-7))*u(1)^2)
  cpO2_T : Fcn  Expr=(25.8911+0.01299*u(1)-0.0000038644*u(1)^2)
  C_p : Outport  VectorParamsAs1DForOutWhenUnconnected=off
  wires:
  T_cool_out/1 -> cpO2_T/1, cpN2_T/1
  cpN2_T/1 -> Product4/1
  N2/1 -> Add1/1, Product4/2
  cpO2_T/1 -> Product5/1
  O2/1 -> Add1/2, Product5/2
  Product4/1 -> Add/1
  Product5/1 -> Add/2
  Add/1 -> Divide/1
  Add1/1 -> Divide/2
  Divide/1 -> C_p/1

== system Hydrogen_platform/Hydrogen_HE/air_out3 ==
  T_cool_out : Inport
  O2 : Inport  Port=2
  N2 : Inport  Port=3
  Add : Sum
  Add1 : Sum
  Divide : Product  Inputs=*/
  Product4 : Product
  Product5 : Product
  cpN2_T : Fcn  Expr=(27.32+(6.226*10^(-3))*u(1)-(9.502*10^(-7))*u(1)^2)
  cpO2_T : Fcn  Expr=(25.8911+0.01299*u(1)-0.0000038644*u(1)^2)
  C_p : Outport  VectorParamsAs1DForOutWhenUnconnected=off
  wires:
  T_cool_out/1 -> cpO2_T/1, cpN2_T/1
  cpN2_T/1 -> Product4/1
  N2/1 -> Add1/1, Product4/2
  cpO2_T/1 -> Product5/1
  O2/1 -> Add1/2, Product5/2
  Product4/1 -> Add/1
  Product5/1 -> Add/2
  Add/1 -> Divide/1
  Add1/1 -> Divide/2
  Divide/1 -> C_p/1

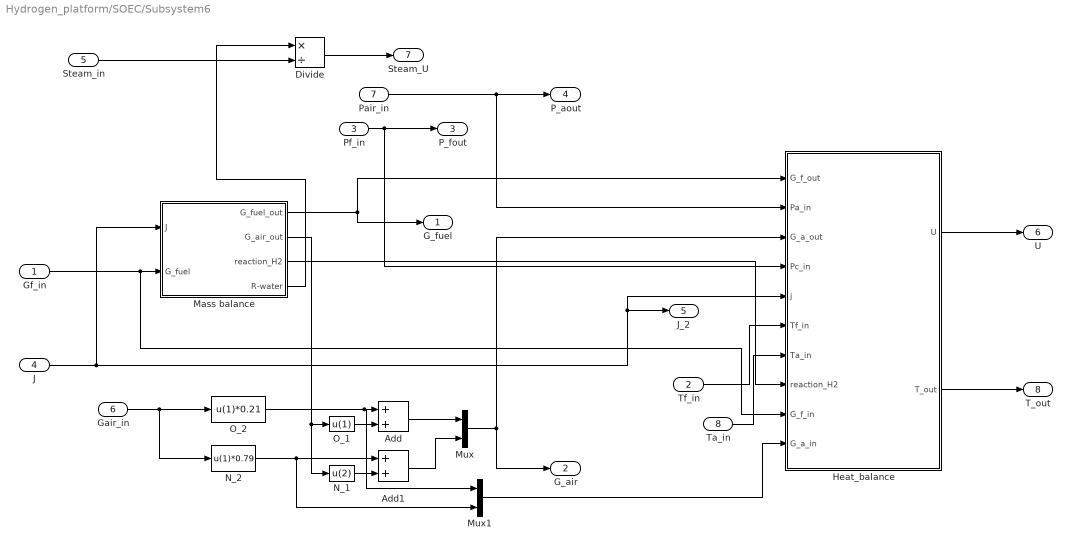
== system Hydrogen_platform/SOEC/Subsystem6 ==
  Gf_in : Inport
  Tf_in : Inport  Port=2
  Pf_in : Inport  Port=3
  J : Inport  Port=4
  Steam_in : Inport  Port=5
  Gair_in : Inport  Port=6
  Pair_in : Inport  Port=7
  Ta_in : Inport  Port=8
  Add : Sum
  Add1 : Sum
  Divide : Product  Inputs=*/
  Heat_balance : Subsystem
  Mass balance : Subsystem
  Mux : Mux  Inputs=2
  Mux1 : Mux  Inputs=2
  N_1 : Fcn  Expr=u(2)
  N_2 : Fcn  Expr=u(1)*0.79
  O_1 : Fcn  Expr=u(1)
  O_2 : Fcn  Expr=u(1)*0.21
  "\tG_fuel" : Outport  VectorParamsAs1DForOutWhenUnconnected=off
  "\tG_air" : Outport  Port=2  VectorParamsAs1DForOutWhenUnconnected=off
  "\tP_fout" : Outport  Port=3  VectorParamsAs1DForOutWhenUnconnected=off
  "\tP_aout" : Outport  Port=4  VectorParamsAs1DForOutWhenUnconnected=off
  J_2 : Outport  Port=5  VectorParamsAs1DForOutWhenUnconnected=off
  U : Outport  Port=6  VectorParamsAs1DForOutWhenUnconnected=off
  Steam_U : Outport  Port=7  VectorParamsAs1DForOutWhenUnconnected=off
  T_out : Outport  Port=8  VectorParamsAs1DForOutWhenUnconnected=off
  wires:
  Gf_in/1 -> Mass balance/2(G_fuel), Heat_balance/9(G_f_in)
  Mass balance/2(G_air_out) -> N_1/1, O_1/1
  Tf_in/1 -> Heat_balance/6(Tf_in)
  J/1 -> Mass balance/1(J), Heat_balance/5(j), J_2/1
  Heat_balance/1(U) -> U/1
  Steam_in/1 -> Divide/2
  Mass balance/1(G_fuel_out) -> "\tG_fuel"/1, Heat_balance/1(G_f_out)
  Divide/1 -> Steam_U/1
  Heat_balance/2(T_out) -> T_out/1
  Mass balance/4(R-water) -> Divide/1
  Gair_in/1 -> N_2/1, O_2/1
  O_2/1 -> Mux1/1, Add/1
  N_2/1 -> Mux1/2, Add1/1
  O_1/1 -> Add/2
  N_1/1 -> Add1/2
  Add/1 -> Mux/1
  Add1/1 -> Mux/2
  Mux/1 -> Heat_balance/3(G_a_out), "\tG_air"/1
  Pf_in/1 -> "\tP_fout"/1, Heat_balance/4(Pc_in)
  Pair_in/1 -> Heat_balance/2(Pa_in), "\tP_aout"/1
  Ta_in/1 -> Heat_balance/7(Ta_in)
  Mass balance/3(reaction_H2) -> Heat_balance/8(reaction_H2)
  Mux1/1 -> Heat_balance/10(G_a_in)

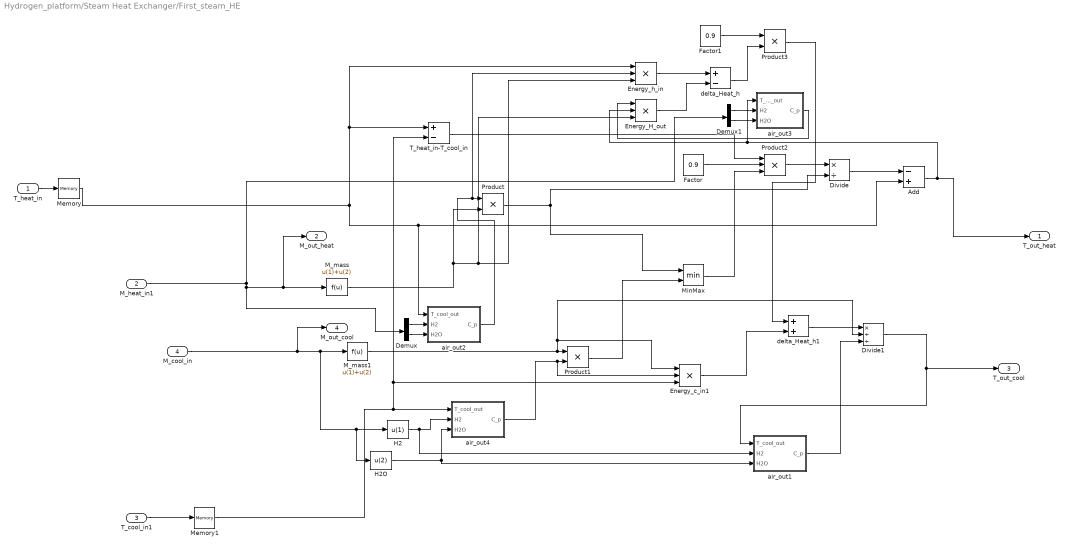
== system Hydrogen_platform/Steam Heat Exchanger/First_steam_HE ==
  T_heat_in : Inport
  M_heat_in1 : Inport  Port=2
  T_cool_in1 : Inport  Port=3
  M_cool_in : Inport  Port=4
  Add : Sum  Inputs=-+
  Demux : Demux  Outputs=2
  Demux1 : Demux  Outputs=2
  Divide : Product  Inputs=*/
  Divide1 : Product  Inputs=*//
  Energy_H_out : Product  Inputs=3
  Energy_c_in1 : Product  Inputs=3
  Energy_h_in : Product  Inputs=3
  Factor : Constant  Value=0.9
  Factor1 : Constant  Value=0.9
  H2 : Fcn  Expr=u(1)
  H2O : Fcn  Expr=u(2)
  M_mass : Fcn  Expr=u(1)+u(2)
  M_mass1 : Fcn  Expr=u(1)+u(2)
  Memory : Memory  InitialCondition=1100
  Memory1 : Memory  InitialCondition=540
  MinMax : MinMax  Inputs=2
  Product : Product
  Product1 : Product
  Product2 : Product  Inputs=3
  Product3 : Product
  T_heat_in-T_cool_in : Sum  Inputs=+-
  air_out1 : Subsystem
  air_out2 : Subsystem
  air_out3 : Subsystem
  air_out4 : Subsystem
  delta_Heat_h : Sum  Inputs=+-
  delta_Heat_h1 : Sum
  T_out_heat : Outport
  M_out_heat : Outport  Port=2
  T_out_cool : Outport  Port=3
  M_out_cool : Outport  Port=4
  wires:
  Product2/1 -> Divide/1
  T_heat_in/1 -> Memory/1
  MinMax/1 -> Product2/3
  M_cool_in/1 -> M_out_cool/1, M_mass1/1, H2O/1, H2/1
  air_out4/1(C_p) -> Energy_c_in1/2, Product1/2
  T_cool_in1/1 -> Memory1/1
  T_heat_in-T_cool_in/1 -> Product2/1
  air_out2/1(C_p) -> Product/1, Energy_h_in/2
  Factor/1 -> Product2/2
  Energy_H_out/1 -> delta_Heat_h/2
  Product1/1 -> MinMax/2
  Product/1 -> MinMax/1, Divide/2
  Add/1 -> T_out_heat/1, air_out3/1(T_cool_out), Energy_H_out/2
  Divide/1 -> Add/1
  Energy_h_in/1 -> delta_Heat_h/1
  Energy_c_in1/1 -> delta_Heat_h1/2
  delta_Heat_h1/1 -> Divide1/1
  air_out1/1(C_p) -> Divide1/3
  Divide1/1 -> air_out1/1(T_cool_out), T_out_cool/1
  delta_Heat_h/1 -> Product3/2
  Product3/1 -> delta_Heat_h1/1
  Factor1/1 -> Product3/1
  M_heat_in1/1 -> Demux/1, M_mass/1, M_out_heat/1, Demux1/1
  Demux/1 -> air_out2/2(H2)
  Demux/2 -> air_out2/3(H2O)
  Demux1/1 -> air_out3/2(H2)
  Demux1/2 -> air_out3/3(H2O)
  air_out3/1(C_p) -> Energy_H_out/1
  H2/1 -> air_out1/2(H2), air_out4/2(H2)
  H2O/1 -> air_out1/3(H2O), air_out4/3(H2O)
  M_mass/1 -> Energy_h_in/3, Energy_H_out/3, Product/2
  M_mass1/1 -> Energy_c_in1/1, Divide1/2, Product1/1
  Memory/1 -> Energy_h_in/1, T_heat_in-T_cool_in/1, air_out2/1(T_cool_out), Add/2
  Memory1/1 -> Energy_c_in1/3, T_heat_in-T_cool_in/2, air_out4/1(T_cool_out)

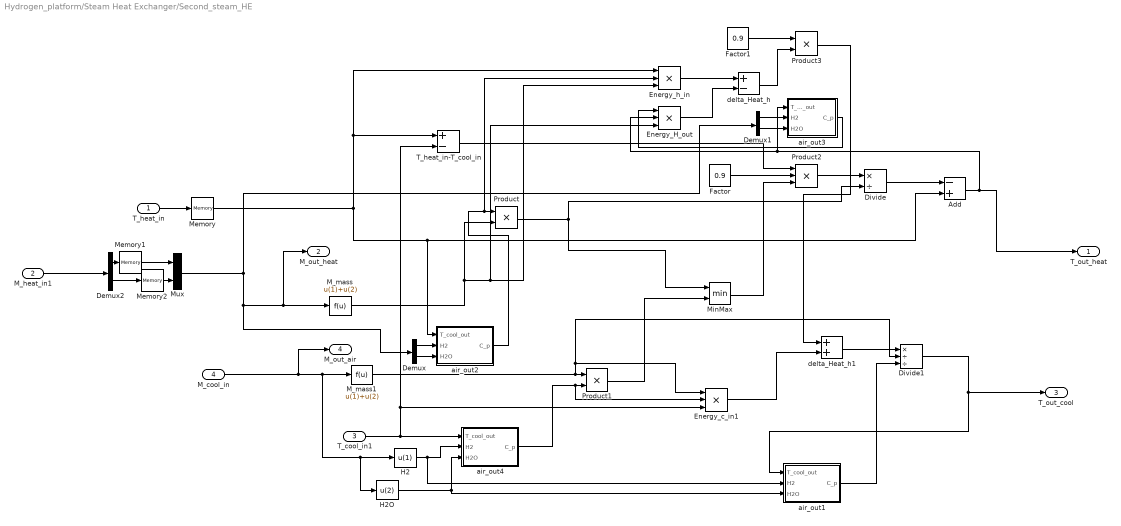
== system Hydrogen_platform/Steam Heat Exchanger/Second_steam_HE ==
  T_heat_in : Inport
  M_heat_in1 : Inport  Port=2
  T_cool_in1 : Inport  Port=3
  M_cool_in : Inport  Port=4
  Add : Sum  Inputs=-+
  Demux : Demux  Outputs=2
  Demux1 : Demux  Outputs=2
  Demux2 : Demux  Outputs=2
  Divide : Product  Inputs=*/
  Divide1 : Product  Inputs=*//
  Energy_H_out : Product  Inputs=3
  Energy_c_in1 : Product  Inputs=3
  Energy_h_in : Product  Inputs=3
  Factor : Constant  Value=0.9
  Factor1 : Constant  Value=0.9
  H2 : Fcn  Expr=u(1)
  H2O : Fcn  Expr=u(2)
  M_mass : Fcn  Expr=u(1)+u(2)
  M_mass1 : Fcn  Expr=u(1)+u(2)
  Memory : Memory  InitialCondition=500
  Memory1 : Memory  InitialCondition=3
  Memory2 : Memory  InitialCondition=1
  MinMax : MinMax  Inputs=2
  Mux : Mux  Inputs=2
  Product : Product
  Product1 : Product
  Product2 : Product  Inputs=3
  Product3 : Product
  T_heat_in-T_cool_in : Sum  Inputs=+-
  air_out1 : Subsystem
  air_out2 : Subsystem
  air_out3 : Subsystem
  air_out4 : Subsystem
  delta_Heat_h : Sum  Inputs=+-
  delta_Heat_h1 : Sum
  T_out_heat : Outport
  M_out_heat : Outport  Port=2
  T_out_cool : Outport  Port=3
  M_out_air : Outport  Port=4
  wires:
  Product2/1 -> Divide/1
  T_heat_in/1 -> Memory/1
  MinMax/1 -> Product2/3
  M_cool_in/1 -> M_out_air/1, M_mass1/1, H2O/1, H2/1
  air_out4/1(C_p) -> Energy_c_in1/2, Product1/2
  T_cool_in1/1 -> Energy_c_in1/3, T_heat_in-T_cool_in/2, air_out4/1(T_cool_out)
  T_heat_in-T_cool_in/1 -> Product2/1
  air_out2/1(C_p) -> Product/1, Energy_h_in/2
  Factor/1 -> Product2/2
  Energy_H_out/1 -> delta_Heat_h/2
  Product1/1 -> MinMax/2
  Product/1 -> MinMax/1, Divide/2
  Add/1 -> air_out3/1(T_cool_out), Energy_H_out/2, T_out_heat/1
  Divide/1 -> Add/1
  Energy_h_in/1 -> delta_Heat_h/1
  Energy_c_in1/1 -> delta_Heat_h1/2
  delta_Heat_h1/1 -> Divide1/1
  air_out1/1(C_p) -> Divide1/3
  Divide1/1 -> air_out1/1(T_cool_out), T_out_cool/1
  delta_Heat_h/1 -> Product3/2
  Product3/1 -> delta_Heat_h1/1
  Factor1/1 -> Product3/1
  Mux/1 -> Demux/1, M_mass/1, M_out_heat/1, Demux1/1
  Demux/1 -> air_out2/2(H2)
  Demux/2 -> air_out2/3(H2O)
  Demux1/1 -> air_out3/2(H2)
  Demux1/2 -> air_out3/3(H2O)
  air_out3/1(C_p) -> Energy_H_out/1
  H2/1 -> air_out1/2(H2), air_out4/2(H2)
  H2O/1 -> air_out1/3(H2O), air_out4/3(H2O)
  M_mass/1 -> Energy_h_in/3, Energy_H_out/3, Product/2
  M_mass1/1 -> Energy_c_in1/1, Divide1/2, Product1/1
  Memory/1 -> Energy_h_in/1, T_heat_in-T_cool_in/1, air_out2/1(T_cool_out), Add/2
  Demux2/2 -> Memory2/1
  Memory2/1 -> Mux/2
  Memory1/1 -> Mux/1
  Demux2/1 -> Memory1/1
  M_heat_in1/1 -> Demux2/1

== system Hydrogen_platform/Air Heat Exchanger/First_Air_HE/air_out ==
  T_cool_out : Inport
  O2 : Inport  Port=2
  N2 : Inport  Port=3
  Add : Sum
  Add1 : Sum
  Divide : Product  Inputs=*/
  Product4 : Product
  Product5 : Product
  cpN2_T : Fcn  Expr=(27.32+(6.226*10^(-3))*u(1)-(9.502*10^(-7))*u(1)^2)
  cpO2_T : Fcn  Expr=(25.8911+0.01299*u(1)-0.0000038644*u(1)^2)
  C_p : Outport  VectorParamsAs1DForOutWhenUnconnected=off
  wires:
  T_cool_out/1 -> cpO2_T/1, cpN2_T/1
  cpN2_T/1 -> Product4/1
  N2/1 -> Add1/1, Product4/2
  cpO2_T/1 -> Product5/1
  O2/1 -> Add1/2, Product5/2
  Product4/1 -> Add/1
  Product5/1 -> Add/2
  Add/1 -> Divide/1
  Add1/1 -> Divide/2
  Divide/1 -> C_p/1

== system Hydrogen_platform/Air Heat Exchanger/First_Air_HE/air_out1 ==
  T_cool_out : Inport
  O2 : Inport  Port=2
  N2 : Inport  Port=3
  Add : Sum
  Add1 : Sum
  Divide : Product  Inputs=*/
  Memory : Memory  InitialCondition=1012
  Product4 : Product
  Product5 : Product
  cpN2_T : Fcn  Expr=(27.32+(6.226*10^(-3))*u(1)-(9.502*10^(-7))*u(1)^2)
  cpO2_T : Fcn  Expr=(25.8911+0.01299*u(1)-0.0000038644*u(1)^2)
  C_p : Outport  VectorParamsAs1DForOutWhenUnconnected=off
  wires:
  T_cool_out/1 -> Memory/1
  cpN2_T/1 -> Product4/1
  N2/1 -> Add1/1, Product4/2
  cpO2_T/1 -> Product5/1
  O2/1 -> Add1/2, Product5/2
  Product4/1 -> Add/1
  Product5/1 -> Add/2
  Add/1 -> Divide/1
  Add1/1 -> Divide/2
  Divide/1 -> C_p/1
  Memory/1 -> cpO2_T/1, cpN2_T/1

== system Hydrogen_platform/Air Heat Exchanger/First_Air_HE/air_out2 ==
  T_cool_out : Inport
  O2 : Inport  Port=2
  N2 : Inport  Port=3
  Add : Sum
  Add1 : Sum
  Divide : Product  Inputs=*/
  Product4 : Product
  Product5 : Product
  cpN2_T : Fcn  Expr=(27.32+(6.226*10^(-3))*u(1)-(9.502*10^(-7))*u(1)^2)
  cpO2_T : Fcn  Expr=(25.8911+0.01299*u(1)-0.0000038644*u(1)^2)
  C_p : Outport  VectorParamsAs1DForOutWhenUnconnected=off
  wires:
  T_cool_out/1 -> cpO2_T/1, cpN2_T/1
  cpN2_T/1 -> Product4/1
  N2/1 -> Add1/1, Product4/2
  cpO2_T/1 -> Product5/1
  O2/1 -> Add1/2, Product5/2
  Product4/1 -> Add/1
  Product5/1 -> Add/2
  Add/1 -> Divide/1
  Add1/1 -> Divide/2
  Divide/1 -> C_p/1

== system Hydrogen_platform/Air Heat Exchanger/First_Air_HE/air_out3 ==
  T_cool_out : Inport
  O2 : Inport  Port=2
  N2 : Inport  Port=3
  Add : Sum
  Add1 : Sum
  Divide : Product  Inputs=*/
  Product4 : Product
  Product5 : Product
  cpN2_T : Fcn  Expr=(27.32+(6.226*10^(-3))*u(1)-(9.502*10^(-7))*u(1)^2)
  cpO2_T : Fcn  Expr=(25.8911+0.01299*u(1)-0.0000038644*u(1)^2)
  C_p : Outport  VectorParamsAs1DForOutWhenUnconnected=off
  wires:
  T_cool_out/1 -> cpO2_T/1, cpN2_T/1
  cpN2_T/1 -> Product4/1
  N2/1 -> Add1/1, Product4/2
  cpO2_T/1 -> Product5/1
  O2/1 -> Add1/2, Product5/2
  Product4/1 -> Add/1
  Product5/1 -> Add/2
  Add/1 -> Divide/1
  Add1/1 -> Divide/2
  Divide/1 -> C_p/1

== system Hydrogen_platform/Air Heat Exchanger/Second_Air_HE/air_out ==
  T_cool_out : Inport
  O2 : Inport  Port=2
  N2 : Inport  Port=3
  Add : Sum
  Add1 : Sum
  Divide : Product  Inputs=*/
  Product4 : Product
  Product5 : Product
  cpN2_T : Fcn  Expr=(27.32+(6.226*10^(-3))*u(1)-(9.502*10^(-7))*u(1)^2)
  cpO2_T : Fcn  Expr=(25.8911+0.01299*u(1)-0.0000038644*u(1)^2)
  C_p : Outport  VectorParamsAs1DForOutWhenUnconnected=off
  wires:
  T_cool_out/1 -> cpO2_T/1, cpN2_T/1
  cpN2_T/1 -> Product4/1
  N2/1 -> Add1/1, Product4/2
  cpO2_T/1 -> Product5/1
  O2/1 -> Add1/2, Product5/2
  Product4/1 -> Add/1
  Product5/1 -> Add/2
  Add/1 -> Divide/1
  Add1/1 -> Divide/2
  Divide/1 -> C_p/1

== system Hydrogen_platform/Air Heat Exchanger/Second_Air_HE/air_out1 ==
  T_cool_out : Inport
  O2 : Inport  Port=2
  N2 : Inport  Port=3
  Add : Sum
  Add1 : Sum
  Divide : Product  Inputs=*/
  Memory : Memory  InitialCondition=700
  Product4 : Product
  Product5 : Product
  cpN2_T : Fcn  Expr=(27.32+(6.226*10^(-3))*u(1)-(9.502*10^(-7))*u(1)^2)
  cpO2_T : Fcn  Expr=(25.8911+0.01299*u(1)-0.0000038644*u(1)^2)
  C_p : Outport  VectorParamsAs1DForOutWhenUnconnected=off
  wires:
  T_cool_out/1 -> Memory/1
  cpN2_T/1 -> Product4/1
  N2/1 -> Add1/1, Product4/2
  cpO2_T/1 -> Product5/1
  O2/1 -> Add1/2, Product5/2
  Product4/1 -> Add/1
  Product5/1 -> Add/2
  Add/1 -> Divide/1
  Add1/1 -> Divide/2
  Divide/1 -> C_p/1
  Memory/1 -> cpO2_T/1, cpN2_T/1

== system Hydrogen_platform/Air Heat Exchanger/Second_Air_HE/air_out2 ==
  T_cool_out : Inport
  O2 : Inport  Port=2
  N2 : Inport  Port=3
  Add : Sum
  Add1 : Sum
  Divide : Product  Inputs=*/
  Product4 : Product
  Product5 : Product
  cpN2_T : Fcn  Expr=(27.32+(6.226*10^(-3))*u(1)-(9.502*10^(-7))*u(1)^2)
  cpO2_T : Fcn  Expr=(25.8911+0.01299*u(1)-0.0000038644*u(1)^2)
  C_p : Outport  VectorParamsAs1DForOutWhenUnconnected=off
  wires:
  T_cool_out/1 -> cpO2_T/1, cpN2_T/1
  cpN2_T/1 -> Product4/1
  N2/1 -> Add1/1, Product4/2
  cpO2_T/1 -> Product5/1
  O2/1 -> Add1/2, Product5/2
  Product4/1 -> Add/1
  Product5/1 -> Add/2
  Add/1 -> Divide/1
  Add1/1 -> Divide/2
  Divide/1 -> C_p/1

== system Hydrogen_platform/Air Heat Exchanger/Second_Air_HE/air_out3 ==
  T_cool_out : Inport
  O2 : Inport  Port=2
  N2 : Inport  Port=3
  Add : Sum
  Add1 : Sum
  Divide : Product  Inputs=*/
  Product4 : Product
  Product5 : Product
  cpN2_T : Fcn  Expr=(27.32+(6.226*10^(-3))*u(1)-(9.502*10^(-7))*u(1)^2)
  cpO2_T : Fcn  Expr=(25.8911+0.01299*u(1)-0.0000038644*u(1)^2)
  C_p : Outport  VectorParamsAs1DForOutWhenUnconnected=off
  wires:
  T_cool_out/1 -> cpO2_T/1, cpN2_T/1
  cpN2_T/1 -> Product4/1
  N2/1 -> Add1/1, Product4/2
  cpO2_T/1 -> Product5/1
  O2/1 -> Add1/2, Product5/2
  Product4/1 -> Add/1
  Product5/1 -> Add/2
  Add/1 -> Divide/1
  Add1/1 -> Divide/2
  Divide/1 -> C_p/1

== system Hydrogen_platform/SOEC/Subsystem6/Heat_balance ==
  G_f_out : Inport
  Pa_in : Inport  Port=2
  G_a_out : Inport  Port=3
  Pc_in : Inport  Port=4
  j : Inport  Port=5
  Tf_in : Inport  Port=6
  Ta_in : Inport  Port=7
  reaction_H2 : Inport  Port=8
  G_f_in : Inport  Port=9
  G_a_in : Inport  Port=10
  Heat : Subsystem
  Memory : Memory  InitialCondition=900
  Scope1 : Scope
  Voltage : Subsystem
  U : Outport  VectorParamsAs1DForOutWhenUnconnected=off
  T_out : Outport  Port=2  VectorParamsAs1DForOutWhenUnconnected=off
  wires:
  Pa_in/1 -> Voltage/2(P_anode_in)
  Pc_in/1 -> Voltage/4(P_cathode_in)
  j/1 -> Voltage/5(j)
  Voltage/1(Uout) -> Scope1/1, U/1
  G_a_out/1 -> Heat/3(G_air_out), Voltage/3(Gair)
  G_f_out/1 -> Heat/2(G_fuel_out), Voltage/1(Ganode_in)
  Tf_in/1 -> Heat/1(T_fuel_in)
  Voltage/2(P_SOEC_con) -> Heat/4(P_in)
  Ta_in/1 -> Heat/5(T_air_in1)
  reaction_H2/1 -> Heat/6(reaction_H2)
  G_f_in/1 -> Heat/7(G_fuel_in)
  G_a_in/1 -> Heat/8(G_air_in)
  Heat/1(Ts) -> Memory/1, T_out/1
  Memory/1 -> Voltage/6(T_in)

== system Hydrogen_platform/SOEC/Subsystem6/Mass balance ==
  J : Inport
  G_fuel : Inport  Port=2
  Add : Sum
  Add1 : Sum  Inputs=+-
  Area : Constant  Value=0.1*0.1
  CO : Fcn  Expr=u(2)
  CO2 : Fcn  Expr=u(3)
  Ch4 : Fcn  Expr=u(1)
  H2O : Fcn  Expr=u(5)
  Mux : Mux  Inputs=5
  Mux1 : Mux  Inputs=2
  N2 : Constant  Value=0  VectorParams1D=off  SampleTime=-1
  O2 : Gain  Gain=0.5
  Rate of Hydarogen : Product  Inputs=**
  Reaction rate : Fcn  Expr=u(1)/2/96485
  h2 : Fcn  Expr=u(4)
  G_fuel_out : Outport
  G_air_out : Outport  Port=2
  reaction_H2 : Outport  Port=3
  R-water : Outport  Port=4
  wires:
  Area/1 -> Rate of Hydarogen/1
  Reaction rate/1 -> Rate of Hydarogen/2
  G_fuel/1 -> H2O/1, h2/1, CO2/1, CO/1, Ch4/1
  Ch4/1 -> Mux/1
  CO/1 -> Mux/2
  CO2/1 -> Mux/3
  h2/1 -> Add/1
  Add/1 -> Mux/4
  Rate of Hydarogen/1 -> R-water/1, reaction_H2/1, Add1/2, Add/2, O2/1
  H2O/1 -> Add1/1
  Add1/1 -> Mux/5
  Mux/1 -> G_fuel_out/1
  N2/1 -> Mux1/2
  O2/1 -> Mux1/1
  Mux1/1 -> G_air_out/1
  J/1 -> Reaction rate/1

== system Hydrogen_platform/Steam Heat Exchanger/First_steam_HE/air_out1 ==
  T_cool_out : Inport
  H2 : Inport  Port=2
  H2O : Inport  Port=3
  Add : Sum
  Add1 : Sum
  Divide : Product  Inputs=*/
  Memory : Memory  InitialCondition=923
  Product4 : Product
  Product5 : Product
  cpH20_T : Fcn  Expr=(30.3794+0.0096212*u(1)-0.0000011848*u(1)^2)
  cpH2_T : Fcn  Expr=(29.08-0.00084*u(1)+0.000002*u(1)^2)
  C_p : Outport  VectorParamsAs1DForOutWhenUnconnected=off
  wires:
  T_cool_out/1 -> Memory/1
  cpH20_T/1 -> Product4/1
  H2O/1 -> Add1/1, Product4/2
  cpH2_T/1 -> Product5/1
  H2/1 -> Add1/2, Product5/2
  Product4/1 -> Add/1
  Product5/1 -> Add/2
  Add/1 -> Divide/1
  Add1/1 -> Divide/2
  Divide/1 -> C_p/1
  Memory/1 -> cpH20_T/1, cpH2_T/1

== system Hydrogen_platform/Steam Heat Exchanger/First_steam_HE/air_out2 ==
  T_cool_out : Inport
  H2 : Inport  Port=2
  H2O : Inport  Port=3
  Add : Sum
  Add1 : Sum
  Divide : Product  Inputs=*/
  Product4 : Product
  Product5 : Product
  cpH20_T : Fcn  Expr=(30.3794+0.0096212*u(1)-0.0000011848*u(1)^2)
  cpH2_T : Fcn  Expr=(29.08-0.00084*u(1)+0.000002*u(1)^2)
  C_p : Outport  VectorParamsAs1DForOutWhenUnconnected=off
  wires:
  T_cool_out/1 -> cpH20_T/1, cpH2_T/1
  cpH20_T/1 -> Product4/1
  H2O/1 -> Add1/1, Product4/2
  cpH2_T/1 -> Product5/1
  H2/1 -> Add1/2, Product5/2
  Product4/1 -> Add/1
  Product5/1 -> Add/2
  Add/1 -> Divide/1
  Add1/1 -> Divide/2
  Divide/1 -> C_p/1

== system Hydrogen_platform/Steam Heat Exchanger/First_steam_HE/air_out3 ==
  T_cool_out : Inport
  H2 : Inport  Port=2
  H2O : Inport  Port=3
  Add : Sum
  Add1 : Sum
  Divide : Product  Inputs=*/
  Product4 : Product
  Product5 : Product
  cpH20_T : Fcn  Expr=(30.3794+0.0096212*u(1)-0.0000011848*u(1)^2)
  cpH2_T : Fcn  Expr=(29.08-0.00084*u(1)+0.000002*u(1)^2)
  C_p : Outport  VectorParamsAs1DForOutWhenUnconnected=off
  wires:
  T_cool_out/1 -> cpH20_T/1, cpH2_T/1
  cpH20_T/1 -> Product4/1
  H2O/1 -> Add1/1, Product4/2
  cpH2_T/1 -> Product5/1
  H2/1 -> Add1/2, Product5/2
  Product4/1 -> Add/1
  Product5/1 -> Add/2
  Add/1 -> Divide/1
  Add1/1 -> Divide/2
  Divide/1 -> C_p/1

== system Hydrogen_platform/Steam Heat Exchanger/First_steam_HE/air_out4 ==
  T_cool_out : Inport
  H2 : Inport  Port=2
  H2O : Inport  Port=3
  Add : Sum
  Add1 : Sum
  Divide : Product  Inputs=*/
  Product4 : Product
  Product5 : Product
  cpH20_T : Fcn  Expr=(30.3794+0.0096212*u(1)-0.0000011848*u(1)^2)
  cpH2_T : Fcn  Expr=(29.08-0.00084*u(1)+0.000002*u(1)^2)
  C_p : Outport  VectorParamsAs1DForOutWhenUnconnected=off
  wires:
  T_cool_out/1 -> cpH20_T/1, cpH2_T/1
  cpH20_T/1 -> Product4/1
  H2O/1 -> Add1/1, Product4/2
  cpH2_T/1 -> Product5/1
  H2/1 -> Add1/2, Product5/2
  Product4/1 -> Add/1
  Product5/1 -> Add/2
  Add/1 -> Divide/1
  Add1/1 -> Divide/2
  Divide/1 -> C_p/1

== system Hydrogen_platform/Steam Heat Exchanger/Second_steam_HE/air_out1 ==
  T_cool_out : Inport
  H2 : Inport  Port=2
  H2O : Inport  Port=3
  Add : Sum
  Add1 : Sum
  Divide : Product  Inputs=*/
  Memory : Memory  InitialCondition=500
  Product4 : Product
  Product5 : Product
  cpH20_T : Fcn  Expr=(30.3794+0.0096212*u(1)-0.0000011848*u(1)^2)
  cpH2_T : Fcn  Expr=(29.08-0.00084*u(1)+0.000002*u(1)^2)
  C_p : Outport  VectorParamsAs1DForOutWhenUnconnected=off
  wires:
  T_cool_out/1 -> Memory/1
  cpH20_T/1 -> Product4/1
  H2O/1 -> Add1/1, Product4/2
  cpH2_T/1 -> Product5/1
  H2/1 -> Add1/2, Product5/2
  Product4/1 -> Add/1
  Product5/1 -> Add/2
  Add/1 -> Divide/1
  Add1/1 -> Divide/2
  Divide/1 -> C_p/1
  Memory/1 -> cpH20_T/1, cpH2_T/1

== system Hydrogen_platform/Steam Heat Exchanger/Second_steam_HE/air_out2 ==
  T_cool_out : Inport
  H2 : Inport  Port=2
  H2O : Inport  Port=3
  Add : Sum
  Add1 : Sum
  Divide : Product  Inputs=*/
  Product4 : Product
  Product5 : Product
  cpH20_T : Fcn  Expr=(30.3794+0.0096212*u(1)-0.0000011848*u(1)^2)
  cpH2_T : Fcn  Expr=(29.08-0.00084*u(1)+0.000002*u(1)^2)
  C_p : Outport  VectorParamsAs1DForOutWhenUnconnected=off
  wires:
  T_cool_out/1 -> cpH20_T/1, cpH2_T/1
  cpH20_T/1 -> Product4/1
  H2O/1 -> Add1/1, Product4/2
  cpH2_T/1 -> Product5/1
  H2/1 -> Add1/2, Product5/2
  Product4/1 -> Add/1
  Product5/1 -> Add/2
  Add/1 -> Divide/1
  Add1/1 -> Divide/2
  Divide/1 -> C_p/1

== system Hydrogen_platform/Steam Heat Exchanger/Second_steam_HE/air_out3 ==
  T_cool_out : Inport
  H2 : Inport  Port=2
  H2O : Inport  Port=3
  Add : Sum
  Add1 : Sum
  Divide : Product  Inputs=*/
  Product4 : Product
  Product5 : Product
  cpH20_T : Fcn  Expr=(30.3794+0.0096212*u(1)-0.0000011848*u(1)^2)
  cpH2_T : Fcn  Expr=(29.08-0.00084*u(1)+0.000002*u(1)^2)
  C_p : Outport  VectorParamsAs1DForOutWhenUnconnected=off
  wires:
  T_cool_out/1 -> cpH20_T/1, cpH2_T/1
  cpH20_T/1 -> Product4/1
  H2O/1 -> Add1/1, Product4/2
  cpH2_T/1 -> Product5/1
  H2/1 -> Add1/2, Product5/2
  Product4/1 -> Add/1
  Product5/1 -> Add/2
  Add/1 -> Divide/1
  Add1/1 -> Divide/2
  Divide/1 -> C_p/1

== system Hydrogen_platform/Steam Heat Exchanger/Second_steam_HE/air_out4 ==
  T_cool_out : Inport
  H2 : Inport  Port=2
  H2O : Inport  Port=3
  Add : Sum
  Add1 : Sum
  Divide : Product  Inputs=*/
  Product4 : Product
  Product5 : Product
  cpH20_T : Fcn  Expr=(30.3794+0.0096212*u(1)-0.0000011848*u(1)^2)
  cpH2_T : Fcn  Expr=(29.08-0.00084*u(1)+0.000002*u(1)^2)
  C_p : Outport  VectorParamsAs1DForOutWhenUnconnected=off
  wires:
  T_cool_out/1 -> cpH20_T/1, cpH2_T/1
  cpH20_T/1 -> Product4/1
  H2O/1 -> Add1/1, Product4/2
  cpH2_T/1 -> Product5/1
  H2/1 -> Add1/2, Product5/2
  Product4/1 -> Add/1
  Product5/1 -> Add/2
  Add/1 -> Divide/1
  Add1/1 -> Divide/2
  Divide/1 -> C_p/1

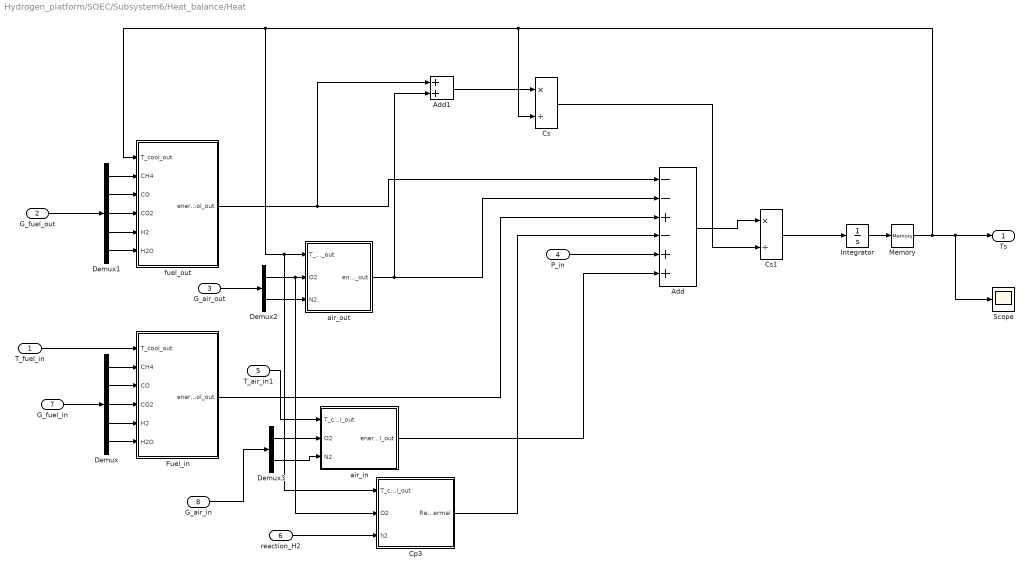
== system Hydrogen_platform/SOEC/Subsystem6/Heat_balance/Heat ==
  T_fuel_in : Inport
  G_fuel_out : Inport  Port=2
  G_air_out : Inport  Port=3
  P_in : Inport  Port=4
  T_air_in1 : Inport  Port=5
  reaction_H2 : Inport  Port=6
  G_fuel_in : Inport  Port=7
  G_air_in : Inport  Port=8
  Add : Sum  Inputs=--+-++
  Add1 : Sum
  Cp3 : Subsystem
  Cs : Product  Inputs=*/
  Cs1 : Product  Inputs=*/
  Demux : Demux  Outputs=5
  Demux1 : Demux  Outputs=5
  Demux2 : Demux  Outputs=2
  Demux3 : Demux  Outputs=2
  Fuel_in : Subsystem
  Integrator : Integrator  InitialCondition=1100
  Memory : Memory  InitialCondition=1000
  Scope : Scope
  air_in : Subsystem
  air_out : Subsystem
  fuel_out : Subsystem
  Ts : Outport
  wires:
  T_fuel_in/1 -> Fuel_in/1(T_cool_out)
  Demux/1 -> Fuel_in/2(CH4)
  Demux/2 -> Fuel_in/3(CO)
  Demux/3 -> Fuel_in/4(CO2)
  Demux/4 -> Fuel_in/5(H2)
  Demux/5 -> Fuel_in/6(H2O)
  G_fuel_out/1 -> Demux1/1
  Demux1/3 -> fuel_out/4(CO2)
  Demux1/4 -> fuel_out/5(H2)
  Demux1/2 -> fuel_out/3(CO)
  Demux1/1 -> fuel_out/2(CH4)
  Demux1/5 -> fuel_out/6(H2O)
  Demux2/2 -> air_out/3(N2)
  G_air_out/1 -> Demux2/1
  fuel_out/1(energy_cool_out) -> Add/1, Add1/1
  air_out/1(energy_cool_out) -> Add1/2, Add/2
  Fuel_in/1(energy_cool_out) -> Add/3
  Cp3/1(Reaction Thermal) -> Add/4
  P_in/1 -> Add/5
  Add1/1 -> Cs/1
  Cs/1 -> Cs1/2
  Demux2/1 -> Cp3/2(O2), air_out/2(O2)
  Integrator/1 -> Memory/1
  Add/1 -> Cs1/1
  Cs1/1 -> Integrator/1
  T_air_in1/1 -> air_in/1(T_cool_out)
  Demux3/1 -> air_in/2(O2)
  Demux3/2 -> air_in/3(N2)
  air_in/1(energy_cool_out) -> Add/6
  reaction_H2/1 -> Cp3/3(h2)
  G_fuel_in/1 -> Demux/1
  G_air_in/1 -> Demux3/1
  Memory/1 -> Cp3/1(T_cool_out), air_out/1(T_cool_out), fuel_out/1(T_cool_out), Cs/2, Scope/1, Ts/1
